simulink model "vhs_fpga_rx_to_sdram_time_share_agc"  (Simulink 7.1)
settings: Solver=FixedStepDiscrete  SolverMode=SingleTasking  StartTime=0.0  StopTime=inf  RelTol=1e-3
values from neighbouring files (symbols this model uses):
  N_FB_RX_frame = 390    [OFDM_Parameter.mat]
  Nfft = 64    [OFDM_Parameter.mat]
  Nguard = 16    [OFDM_Parameter.mat]
  Nofdm = 130    [OFDM_Parameter.mat]
libraries: xbsIndex_r4 x181, vhsadac_common_ob_fpgalib_v1_2_0 x17, misc_tools_fpgalib_v1_0_0 x2, rffe_fpgalib_v1_1_0 x1, rtdex_fpgalib_v1_1_0 x1
(part 2 of 2)

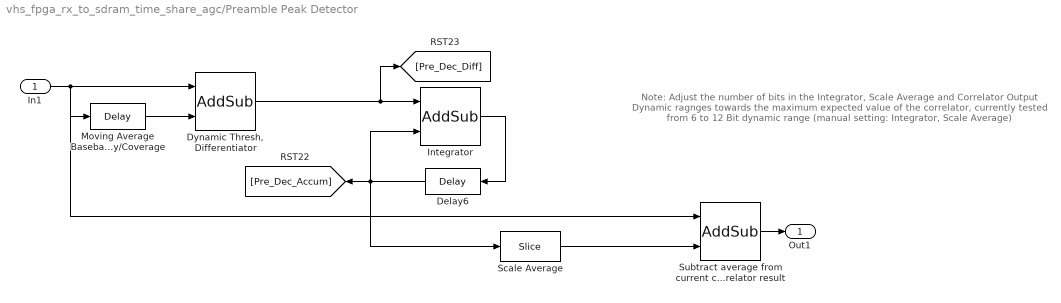
== system vhs_fpga_rx_to_sdram_time_share_agc/Preamble Peak Detector ==
  note: Note: Adjust the number of bits in the Integrator, Scale Average and Correlator Output Dynamic ragnges
      |  towards the maximum expected value of the correlator, currently tested from 6 to 12 Bit dynamic range
      |  (manual setting: Integrator, Scale Average)
  In1 : Inport
  Delay6 : xbsIndex_r4/Delay  Orientation=left  en=off  latency=1  dbl_ovrd=off  reg_retiming=off  block_type=delay
  "Dynamic Thresh, Differentiator" : xbsIndex_r4/AddSub  mode=Subtraction  use_carryin=off  use_carryout=off  en=off  latency=0  precision=Full  arith_type=Unsigned  n_bits=16  bin_pt=14  quantization=Truncate  overflow=Wrap  dbl_ovrd=off  use_behavioral_HDL=off  pipelined=off  use_rpm=on  hw_selection=Fabric  block_type=addsub
      settings: block_version=10.1.3
  Integrator : xbsIndex_r4/AddSub  mode=Addition  use_carryin=off  use_carryout=off  en=off  latency=0  precision=User Defined  arith_type="Signed  (2's comp)"  n_bits=23  bin_pt=0  quantization=Truncate  overflow=Saturate  dbl_ovrd=off  use_behavioral_HDL=off  pipelined=off  use_rpm=on  hw_selection=Fabric  block_type=addsub
      settings: block_version=10.1.3
  Moving Average Baseband (20MHz) Delay/Coverage : xbsIndex_r4/Delay  en=off  latency=32  dbl_ovrd=off  reg_retiming=off  block_type=delay
  Scale Average : xbsIndex_r4/Slice  nbits=16  boolean_output=off  mode=Upper Bit Location + Width  bit1=-7  base1=MSB of Input  bit0=0  base0=LSB of Input  dbl_ovrd=off  block_type=slice
      settings: infoedit="Extracts a given range of bits from each input sample and presents it at the output.  The output type is ordinarily unsigned with binary point at zero, but can be Boolean when the slice is one bit wide.<P><P>Hardware notes: In hardware this block costs nothing."  block_version=10.1.3
  Subtract average from current correlator result : xbsIndex_r4/AddSub  mode=Subtraction  use_carryin=off  use_carryout=off  en=off  latency=0  precision=Full  arith_type=Unsigned  n_bits=16  bin_pt=14  quantization=Truncate  overflow=Wrap  dbl_ovrd=off  use_behavioral_HDL=off  pipelined=off  use_rpm=on  hw_selection=Fabric  block_type=addsub
      settings: block_version=10.1.3
  Out1 : Outport
  wires:
  Moving Average Baseband (20MHz) Delay/Coverage/1 -> "Dynamic Thresh, Differentiator"/2
  "Dynamic Thresh, Differentiator"/1 -> Integrator/1, [Pre_Dec_Diff]
  Integrator/1 -> Delay6/1
  Delay6/1 -> Integrator/2, [Pre_Dec_Accum], Scale Average/1
  Scale Average/1 -> Subtract average from current correlator result/2
  In1/1 -> Moving Average Baseband (20MHz) Delay/Coverage/1, Subtract average from current correlator result/1, "Dynamic Thresh, Differentiator"/1
  Subtract average from current correlator result/1 -> Out1/1

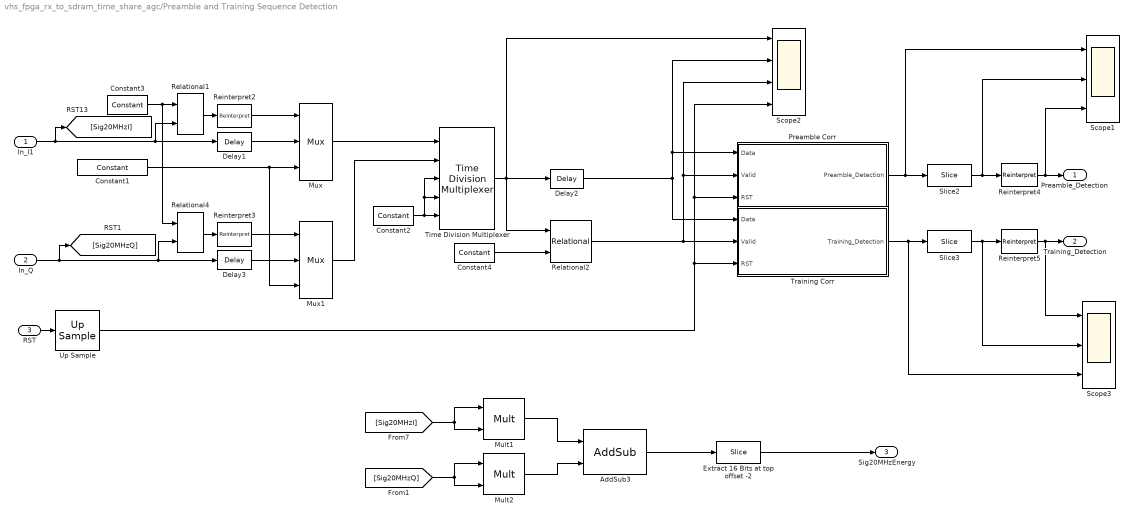
== system vhs_fpga_rx_to_sdram_time_share_agc/Preamble and Training Sequence Detection ==
  In_I1 : Inport  OutDataType=sfix(16)  OutScaling=2^0
  In_Q : Inport  Port=2  OutDataType=sfix(16)  OutScaling=2^0
  RST : Inport  Port=3  OutDataType=sfix(16)  OutScaling=2^0
  "   Extract 16 Bits at top offset -2" : xbsIndex_r4/Slice  nbits=16  boolean_output=off  mode=Upper Bit Location + Width  bit1=-2  base1=MSB of Input  bit0=0  base0=LSB of Input  dbl_ovrd=off  block_type=slice
      settings: infoedit="Extracts a given range of bits from each input sample and presents it at the output.  The output type is ordinarily unsigned with binary point at zero, but can be Boolean when the slice is one bit wide.<P><P>Hardware notes: In hardware this block costs nothing."  block_version=10.1.3
  AddSub3 : xbsIndex_r4/AddSub  mode=Addition  use_carryin=off  use_carryout=off  en=off  latency=1  precision=Full  arith_type=Unsigned  n_bits=16  bin_pt=14  quantization=Truncate  overflow=Wrap  dbl_ovrd=off  use_behavioral_HDL=off  pipelined=off  use_rpm=on  hw_selection=Fabric  block_type=addsub
      settings: block_version=10.1.3
  Constant1 : xbsIndex_r4/Constant  arith_type=Signed (2's comp)  const=1  n_bits=14  bin_pt=0  explicit_period=on  period=5  equ=P=C  opselect=C  inp2=PCIN>>17  opr=+  inp1=P  carry=CIN  dbl_ovrd=off  block_type=constant
  Constant2 : xbsIndex_r4/Constant  arith_type=Signed (2's comp)  const=0  n_bits=14  bin_pt=0  explicit_period=on  period=5  equ=P=C  opselect=C  inp2=PCIN>>17  opr=+  inp1=P  carry=CIN  dbl_ovrd=off  block_type=constant
  Constant3 : xbsIndex_r4/Constant  arith_type=Signed (2's comp)  const=0  n_bits=14  bin_pt=13  explicit_period=on  period=5  equ=P=C  opselect=C  inp2=PCIN>>17  opr=+  inp1=P  carry=CIN  dbl_ovrd=off  block_type=constant
  Constant4 : xbsIndex_r4/Constant  arith_type=Unsigned  const=0  n_bits=2  bin_pt=0  explicit_period=on  period=1  equ=P=C  opselect=C  inp2=PCIN>>17  opr=+  inp1=P  carry=CIN  dbl_ovrd=off  block_type=constant
  Delay1 : xbsIndex_r4/Delay  en=off  latency=1  dbl_ovrd=off  reg_retiming=off  block_type=delay
  Delay2 : xbsIndex_r4/Delay  en=off  latency=1  dbl_ovrd=off  reg_retiming=off  block_type=delay
  Delay3 : xbsIndex_r4/Delay  en=off  latency=1  dbl_ovrd=off  reg_retiming=off  block_type=delay
  Mult1 : xbsIndex_r4/Mult  precision=Full  arith_type="Signed  (2's comp)"  n_bits=16  bin_pt=14  quantization=Truncate  overflow=Wrap  en=off  latency=3  dbl_ovrd=off  use_behavioral_HDL=off  use_embedded=on  opt=Speed  optimum_pipeline=off  pipeline=on  use_rpm=on  placement_style=Triangular  block_type=mult
      settings: infoedit=Hardware notes: To use the internal pipeline stage of the dedicated multiplier you must select 'Pipeline for maximum performance'.  block_version=10.1.3
  Mult2 : xbsIndex_r4/Mult  precision=Full  arith_type="Signed  (2's comp)"  n_bits=16  bin_pt=14  quantization=Truncate  overflow=Wrap  en=off  latency=3  dbl_ovrd=off  use_behavioral_HDL=off  use_embedded=on  opt=Speed  optimum_pipeline=off  pipeline=on  use_rpm=on  placement_style=Triangular  block_type=mult
      settings: infoedit=Hardware notes: To use the internal pipeline stage of the dedicated multiplier you must select 'Pipeline for maximum performance'.  block_version=10.1.3
  Mux : xbsIndex_r4/Mux  inputs=2  en=off  latency=0  precision=Full  arith_type=Unsigned  n_bits=16  bin_pt=14  quantization=Truncate  overflow=Wrap  dbl_ovrd=off  block_type=mux
  Mux1 : xbsIndex_r4/Mux  inputs=2  en=off  latency=0  precision=Full  arith_type=Unsigned  n_bits=16  bin_pt=14  quantization=Truncate  overflow=Wrap  dbl_ovrd=off  block_type=mux
  Preamble Corr : Subsystem
  Reinterpret{2..5} (4 alike) : xbsIndex_r4/Reinterpret  force_arith_type=on  arith_type=Unsigned  force_bin_pt=on  bin_pt=0  block_type=reinterpret
      settings: infoedit="Changes signal type without altering the binary representation.   You can changed the signal between signed and unsigned, and relocate the binary point.<P><P>Hardware notes: In hardware this block costs nothing.<P><P>Example:  Suppose the input is 6 bits wide, signed, with 2 fractional bits, and the output is forced to unsigned with 0 fractional bits.  Then an input of -2.0 (1110.00 in binary 2's complement) becomes an output of 56 (111000 in binary)."  block_version=10.1.3
  Relational1 : xbsIndex_r4/Relational  mode=a=b  en=off  latency=1  dbl_ovrd=off  block_type=relational
      settings: block_version=10.1.3
  Relational2 : xbsIndex_r4/Relational  mode=a!=b  en=off  latency=1  dbl_ovrd=off  block_type=relational
      settings: block_version=10.1.3
  Relational4 : xbsIndex_r4/Relational  mode=a=b  en=off  latency=1  dbl_ovrd=off  block_type=relational
      settings: block_version=10.1.3
  Scope1 : Scope  NumInputPorts=3
      settings: YMin=-5~-5~-5  YMax=5~5~5  SaveName=ScopeData4  MaxDataPoints=500000  SampleInput=on
  Scope2 : Scope  NumInputPorts=4
      settings: YMin=-5~-5~-5~-5  YMax=5~5~5~5  SaveName=ScopeData3  MaxDataPoints=500000
  Scope3 : Scope  NumInputPorts=3
      settings: YMin=-5~-5~-5  YMax=5~5~5  SaveName=ScopeData5  MaxDataPoints=500000  SampleInput=on
  Slice2 : xbsIndex_r4/Slice  nbits=16  boolean_output=off  mode=Upper Bit Location + Width  bit1=-8  base1=MSB of Input  bit0=0  base0=LSB of Input  dbl_ovrd=off  block_type=slice
      settings: infoedit="Extracts a given range of bits from each input sample and presents it at the output.  The output type is ordinarily unsigned with binary point at zero, but can be Boolean when the slice is one bit wide.<P><P>Hardware notes: In hardware this block costs nothing."  block_version=10.1.3
  Slice3 : xbsIndex_r4/Slice  nbits=16  boolean_output=off  mode=Upper Bit Location + Width  bit1=-8  base1=MSB of Input  bit0=0  base0=LSB of Input  dbl_ovrd=off  block_type=slice
      settings: infoedit="Extracts a given range of bits from each input sample and presents it at the output.  The output type is ordinarily unsigned with binary point at zero, but can be Boolean when the slice is one bit wide.<P><P>Hardware notes: In hardware this block costs nothing."  block_version=10.1.3
  Time Division Multiplexer : xbsIndex_r4/Time Division Multiplexer  inputs=5  vin=off  dbl_ovrd=off  explicit_period=off  period=1  block_type=tdm
      settings: infoedit="Multiple inputs are sampled and  presented serially at the output."  block_version=10.1.3
  Training Corr : Subsystem
  Up Sample : xbsIndex_r4/Up Sample  sample_ratio=5  copy_samples=on  dbl_ovrd=off  block_type=usamp
      settings: infoedit="Up samples input data.  Inserted values  can be zeros or copies of the most recent input sample.<P><P>Hardware notes: No hardware is needed if inserted values are copies of the input sample; otherwise, a mux and single bit flip-flop are used."  block_version=10.1.3
  Preamble_Detection : Outport  OutDataType=sfix(16)  OutScaling=2^0
  Training_Detection : Outport  Port=2  OutDataType=sfix(16)  OutScaling=2^0
  Sig20MHzEnergy : Outport  Port=3  OutDataType=sfix(16)  OutScaling=2^0
  wires:
  Preamble Corr/1(Preamble_Detection) -> Slice2/1, Scope1/1
  Training Corr/1(Training_Detection) -> Slice3/1, Scope3/3
  Time Division Multiplexer/1 -> Delay2/1, Scope2/1, Relational2/1
  Constant2/1 -> Time Division Multiplexer/5, Time Division Multiplexer/3, Time Division Multiplexer/4
  In_Q/1 -> Relational4/2, Delay3/1, [Sig20MHzQ]
  In_I1/1 -> Relational1/2, Delay1/1, [Sig20MHzI]
  Constant4/1 -> Relational2/2
  RST/1 -> Up Sample/1
  Delay2/1 -> Training Corr/1(Data), Preamble Corr/1(Data), Scope2/2
  Up Sample/1 -> Training Corr/3(RST), Preamble Corr/3(RST), Scope2/4
  Relational2/1 -> Training Corr/2(Valid), Preamble Corr/2(Valid), Scope2/3
  Mux/1 -> Time Division Multiplexer/1
  Mux1/1 -> Time Division Multiplexer/2
  Constant1/1 -> Mux/3, Mux1/3
  Constant3/1 -> Relational1/1, Relational4/1
  Relational1/1 -> Reinterpret2/1
  Relational4/1 -> Reinterpret3/1
  Reinterpret2/1 -> Mux/1
  Reinterpret3/1 -> Mux1/1
  Delay1/1 -> Mux/2
  Delay3/1 -> Mux1/2
  Slice2/1 -> Reinterpret4/1, Scope1/2
  Slice3/1 -> Reinterpret5/1, Scope3/2
  Reinterpret4/1 -> Preamble_Detection/1, Scope1/3
  Reinterpret5/1 -> Training_Detection/1, Scope3/1
  [Sig20MHzI] -> Mult1/1, Mult1/2
  [Sig20MHzQ] -> Mult2/2, Mult2/1
  Mult1/1 -> AddSub3/1
  Mult2/1 -> AddSub3/2
  AddSub3/1 -> "   Extract 16 Bits at top offset -2"/1
  "   Extract 16 Bits at top offset -2"/1 -> Sig20MHzEnergy/1

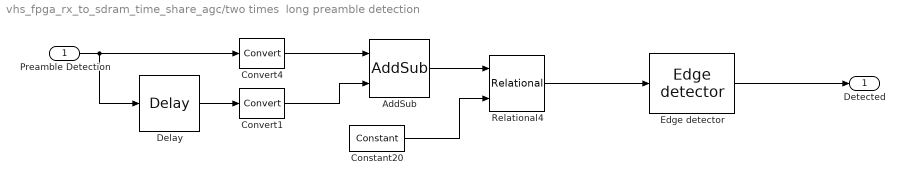
== system vhs_fpga_rx_to_sdram_time_share_agc/two times  long preamble detection ==
  Preamble Detection : Inport  OutDataType=sfix(16)  OutScaling=2^0
  AddSub : xbsIndex_r4/AddSub  mode=Addition  use_carryin=off  use_carryout=off  en=off  latency=0  precision=Full  arith_type=Unsigned  n_bits=16  bin_pt=14  quantization=Truncate  overflow=Wrap  dbl_ovrd=off  use_behavioral_HDL=off  pipelined=off  use_rpm=on  hw_selection=Fabric  block_type=addsub
      settings: block_version=9.2.00
  Constant20 : xbsIndex_r4/Constant  arith_type=Signed (2's comp)  const=2  n_bits=3  bin_pt=0  explicit_period=on  period=5  equ=P=C  opselect=C  inp2=PCIN>>17  opr=+  inp1=P  carry=CIN  dbl_ovrd=off  block_type=constant
      settings: block_version=9.2.00
  Convert1 : xbsIndex_r4/Convert  arith_type="Signed  (2's comp)"  n_bits=3  bin_pt=0  quantization=Truncate  overflow=Wrap  latency=0  dbl_ovrd=off  pipeline=off  block_type=convert
      settings: block_version=9.2.00
  Convert4 : xbsIndex_r4/Convert  arith_type="Signed  (2's comp)"  n_bits=3  bin_pt=0  quantization=Truncate  overflow=Wrap  latency=0  dbl_ovrd=off  pipeline=off  block_type=convert
      settings: block_version=9.2.00
  Delay : xbsIndex_r4/Delay  en=off  latency=(Nfft+Nguard)  dbl_ovrd=off  reg_retiming=off  block_type=delay
      settings: block_version=9.2.00
  Edge detector : misc_tools_fpgalib_v1_0_0/Edge detector  Tag=LYR_FPGA_MISC_EDGE_DETECTOR  Description=Lyrtech block  SystemSampleTime=-1  edge_detect=Rising  and_latency=0
  Relational4 : xbsIndex_r4/Relational  mode=a=b  en=off  latency=1  dbl_ovrd=off  block_type=relational
      settings: block_version=9.2.00
  Detected : Outport  OutDataType=sfix(16)  OutScaling=2^0
  wires:
  AddSub/1 -> Relational4/1
  Constant20/1 -> Relational4/2
  Convert4/1 -> AddSub/1
  Preamble Detection/1 -> Convert4/1, Delay/1
  Convert1/1 -> AddSub/2
  Delay/1 -> Convert1/1
  Relational4/1 -> Edge detector/1
  Edge detector/1 -> Detected/1

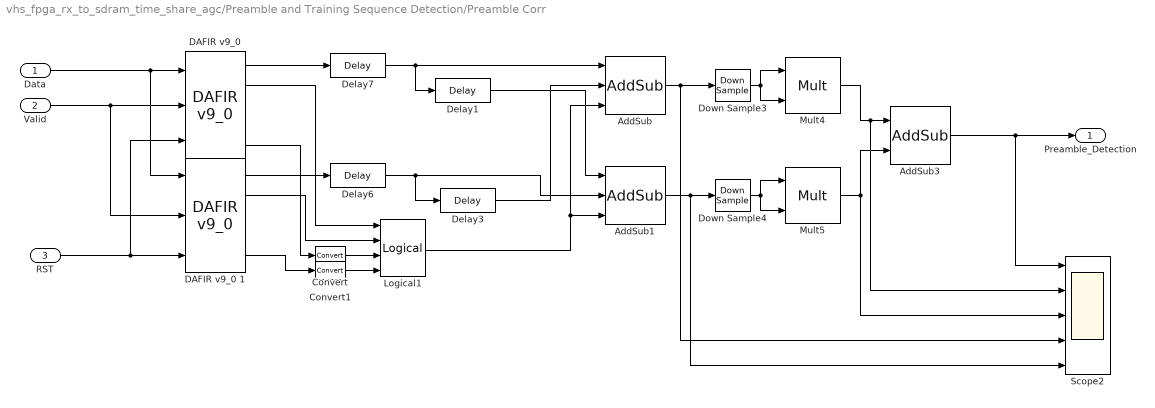
== system vhs_fpga_rx_to_sdram_time_share_agc/Preamble and Training Sequence Detection/Preamble Corr ==
  Data : Inport  OutDataType=sfix(16)  OutScaling=2^0
  Valid : Inport  Port=2  OutDataType=sfix(16)  OutScaling=2^0
  RST : Inport  Port=3  OutDataType=sfix(16)  OutScaling=2^0
  AddSub : xbsIndex_r4/AddSub  mode=Addition  use_carryin=off  use_carryout=off  en=on  latency=1  precision=Full  arith_type=Unsigned  n_bits=16  bin_pt=14  quantization=Truncate  overflow=Wrap  dbl_ovrd=off  use_behavioral_HDL=off  pipelined=off  use_rpm=on  hw_selection=Fabric  block_type=addsub
      settings: block_version=10.1.3
  AddSub1 : xbsIndex_r4/AddSub  mode=Subtraction  use_carryin=off  use_carryout=off  en=on  latency=1  precision=Full  arith_type=Unsigned  n_bits=16  bin_pt=14  quantization=Truncate  overflow=Wrap  dbl_ovrd=off  use_behavioral_HDL=off  pipelined=off  use_rpm=on  hw_selection=Fabric  block_type=addsub
      settings: block_version=10.1.3
  AddSub3 : xbsIndex_r4/AddSub  mode=Addition  use_carryin=off  use_carryout=off  en=off  latency=1  precision=Full  arith_type=Unsigned  n_bits=16  bin_pt=14  quantization=Truncate  overflow=Wrap  dbl_ovrd=off  use_behavioral_HDL=off  pipelined=off  use_rpm=on  hw_selection=Fabric  block_type=addsub
      settings: block_version=10.1.3
  Convert : xbsIndex_r4/Convert  arith_type=Boolean  n_bits=16  bin_pt=14  quantization=Truncate  overflow=Wrap  latency=0  dbl_ovrd=off  pipeline=off  block_type=convert
      settings: block_version=10.1.3
  Convert1 : xbsIndex_r4/Convert  arith_type=Boolean  n_bits=16  bin_pt=14  quantization=Truncate  overflow=Wrap  latency=0  dbl_ovrd=off  pipeline=off  block_type=convert
      settings: block_version=10.1.3
  "DAFIR v9_0 " : xbsIndex_r4/DAFIR v9_0   coef=2^8 * real( conj([(longPreamble_time(end:-1:end-Nguard+1)) (longPreamble_time(end:-1:1))]) )  structure=Inferred from Coefficients  coef_n_bits=10  coef_bin_pt=0  over_sample=1  reload=off  valids=on  rst=on  latency=11  num_channels=2  serial_input=on  polyphase_behavior="Single Rate:  sample in - sample out"  dbl_ovrd=off  explicit_period=off  period=1  use_isim=0  block_type=fir
      settings: infoedit="Hardware notes: Implemented using distributed arithmetic (DA).  The hardware over sampling rate determines the degree of parallelism.  A rate of one produces a fully parallel DA filter.  A rate of n (resp., n+1) for an n-bit input signal produces a fully serial implementation for a non-symmetric (resp., symmetric) impulse response.  Intermediate values produce implementations with intermediate levels of parallelism."  block_version=10.1.3
  DAFIR v9_0 1 : xbsIndex_r4/DAFIR v9_0   coef=2^8 * imag( conj([(longPreamble_time(end:-1:end-Nguard+1)) (longPreamble_time(end:-1:1))]) )  structure=Inferred from Coefficients  coef_n_bits=10  coef_bin_pt=0  over_sample=1  reload=off  valids=on  rst=on  latency=11  num_channels=2  serial_input=on  polyphase_behavior="Single Rate:  sample in - sample out"  dbl_ovrd=off  explicit_period=off  period=1  use_isim=0  block_type=fir
      settings: infoedit="Hardware notes: Implemented using distributed arithmetic (DA).  The hardware over sampling rate determines the degree of parallelism.  A rate of one produces a fully parallel DA filter.  A rate of n (resp., n+1) for an n-bit input signal produces a fully serial implementation for a non-symmetric (resp., symmetric) impulse response.  Intermediate values produce implementations with intermediate levels of parallelism."  block_version=10.1.3
  Delay{1,3,6..7} (4 alike) : xbsIndex_r4/Delay  en=off  latency=1  dbl_ovrd=off  reg_retiming=off  block_type=delay
  Down Sample3 : xbsIndex_r4/Down Sample  sample_ratio=5  sample_phase="Last Value of Frame  (most efficient)"  en=off  latency=1  dbl_ovrd=off  block_type=dsamp
      settings: block_version=10.1.3
  Down Sample4 : xbsIndex_r4/Down Sample  sample_ratio=5  sample_phase="Last Value of Frame  (most efficient)"  en=off  latency=1  dbl_ovrd=off  block_type=dsamp
      settings: block_version=10.1.3
  Logical1 : xbsIndex_r4/Logical  logical_function=AND  inputs=4  en=off  latency=1  precision=Full  arith_type=Unsigned  n_bits=16  bin_pt=0  align_bp=on  dbl_ovrd=off  block_type=logical
  Mult4 : xbsIndex_r4/Mult  precision=Full  arith_type="Signed  (2's comp)"  n_bits=16  bin_pt=14  quantization=Truncate  overflow=Wrap  en=off  latency=3  dbl_ovrd=off  use_behavioral_HDL=off  use_embedded=on  opt=Speed  optimum_pipeline=off  pipeline=on  use_rpm=on  placement_style=Triangular  block_type=mult
      settings: infoedit=Hardware notes: To use the internal pipeline stage of the dedicated multiplier you must select 'Pipeline for maximum performance'.  block_version=10.1.3
  Mult5 : xbsIndex_r4/Mult  precision=Full  arith_type="Signed  (2's comp)"  n_bits=16  bin_pt=14  quantization=Truncate  overflow=Wrap  en=off  latency=3  dbl_ovrd=off  use_behavioral_HDL=off  use_embedded=on  opt=Speed  optimum_pipeline=off  pipeline=on  use_rpm=on  placement_style=Triangular  block_type=mult
      settings: infoedit=Hardware notes: To use the internal pipeline stage of the dedicated multiplier you must select 'Pipeline for maximum performance'.  block_version=10.1.3
  Scope2 : Scope  NumInputPorts=5
      settings: YMin=-5~-5~-5~-5~-5  YMax=5~5~5~5~5  MaxDataPoints=500000
  Preamble_Detection : Outport  OutDataType=sfix(16)  OutScaling=2^0
  wires:
  "DAFIR v9_0 "/2 -> Logical1/1
  DAFIR v9_0 1/2 -> Logical1/2
  "DAFIR v9_0 "/1 -> Delay7/1
  DAFIR v9_0 1/1 -> Delay6/1
  Delay7/1 -> Delay1/1, AddSub/1
  Delay6/1 -> Delay3/1, AddSub1/2
  Delay3/1 -> AddSub/2
  Logical1/1 -> AddSub1/3, AddSub/3
  "DAFIR v9_0 "/5 -> Convert/1
  DAFIR v9_0 1/5 -> Convert1/1
  Convert/1 -> Logical1/3
  Convert1/1 -> Logical1/4
  Valid/1 -> DAFIR v9_0 1/2, "DAFIR v9_0 "/2
  Data/1 -> "DAFIR v9_0 "/1, DAFIR v9_0 1/1
  RST/1 -> "DAFIR v9_0 "/3, DAFIR v9_0 1/3
  Delay1/1 -> AddSub1/1
  AddSub3/1 -> Preamble_Detection/1, Scope2/1
  AddSub/1 -> Scope2/4, Down Sample3/1
  AddSub1/1 -> Down Sample4/1, Scope2/5
  Down Sample3/1 -> Mult4/1, Mult4/2
  Down Sample4/1 -> Mult5/1, Mult5/2
  Mult4/1 -> AddSub3/1, Scope2/2
  Mult5/1 -> AddSub3/2, Scope2/3

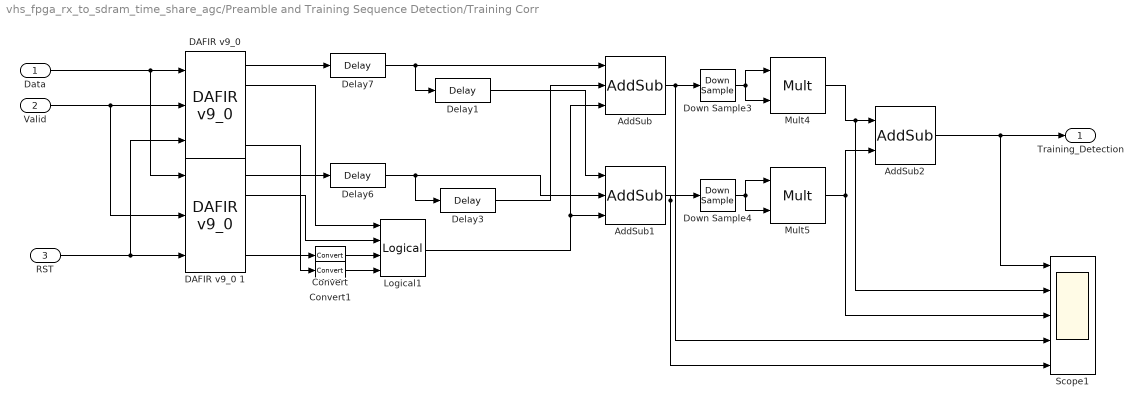
== system vhs_fpga_rx_to_sdram_time_share_agc/Preamble and Training Sequence Detection/Training Corr ==
  Data : Inport  OutDataType=sfix(16)  OutScaling=2^0
  Valid : Inport  Port=2  OutDataType=sfix(16)  OutScaling=2^0
  RST : Inport  Port=3  OutDataType=sfix(16)  OutScaling=2^0
  AddSub : xbsIndex_r4/AddSub  mode=Addition  use_carryin=off  use_carryout=off  en=on  latency=1  precision=Full  arith_type=Unsigned  n_bits=16  bin_pt=14  quantization=Truncate  overflow=Wrap  dbl_ovrd=off  use_behavioral_HDL=off  pipelined=off  use_rpm=on  hw_selection=Fabric  block_type=addsub
      settings: block_version=10.1.3
  AddSub1 : xbsIndex_r4/AddSub  mode=Subtraction  use_carryin=off  use_carryout=off  en=on  latency=1  precision=Full  arith_type=Unsigned  n_bits=16  bin_pt=14  quantization=Truncate  overflow=Wrap  dbl_ovrd=off  use_behavioral_HDL=off  pipelined=off  use_rpm=on  hw_selection=Fabric  block_type=addsub
      settings: block_version=10.1.3
  AddSub2 : xbsIndex_r4/AddSub  mode=Addition  use_carryin=off  use_carryout=off  en=off  latency=1  precision=Full  arith_type=Unsigned  n_bits=16  bin_pt=14  quantization=Truncate  overflow=Wrap  dbl_ovrd=off  use_behavioral_HDL=off  pipelined=off  use_rpm=on  hw_selection=Fabric  block_type=addsub
      settings: block_version=10.1.3
  Convert : xbsIndex_r4/Convert  arith_type=Boolean  n_bits=16  bin_pt=14  quantization=Truncate  overflow=Wrap  latency=0  dbl_ovrd=off  pipeline=off  block_type=convert
      settings: block_version=10.1.3
  Convert1 : xbsIndex_r4/Convert  arith_type=Boolean  n_bits=16  bin_pt=14  quantization=Truncate  overflow=Wrap  latency=0  dbl_ovrd=off  pipeline=off  block_type=convert
      settings: block_version=10.1.3
  "DAFIR v9_0 " : xbsIndex_r4/DAFIR v9_0   coef=2^7 * real( conj([(training_time(end:-1:end-Nguard+1)) (training_time(end:-1:1))]) )  structure=Inferred from Coefficients  coef_n_bits=10  coef_bin_pt=0  over_sample=1  reload=off  valids=on  rst=on  latency=11  num_channels=2  serial_input=on  polyphase_behavior="Single Rate:  sample in - sample out"  dbl_ovrd=off  explicit_period=off  period=1  use_isim=0  block_type=fir
      settings: infoedit="Hardware notes: Implemented using distributed arithmetic (DA).  The hardware over sampling rate determines the degree of parallelism.  A rate of one produces a fully parallel DA filter.  A rate of n (resp., n+1) for an n-bit input signal produces a fully serial implementation for a non-symmetric (resp., symmetric) impulse response.  Intermediate values produce implementations with intermediate levels of parallelism."  block_version=10.1.3
  DAFIR v9_0 1 : xbsIndex_r4/DAFIR v9_0   coef=2^7 * imag( conj([(training_time(end:-1:end-Nguard+1)) (training_time(end:-1:1))]) )  structure=Inferred from Coefficients  coef_n_bits=10  coef_bin_pt=0  over_sample=1  reload=off  valids=on  rst=on  latency=11  num_channels=2  serial_input=on  polyphase_behavior="Single Rate:  sample in - sample out"  dbl_ovrd=off  explicit_period=off  period=1  use_isim=0  block_type=fir
      settings: infoedit="Hardware notes: Implemented using distributed arithmetic (DA).  The hardware over sampling rate determines the degree of parallelism.  A rate of one produces a fully parallel DA filter.  A rate of n (resp., n+1) for an n-bit input signal produces a fully serial implementation for a non-symmetric (resp., symmetric) impulse response.  Intermediate values produce implementations with intermediate levels of parallelism."  block_version=10.1.3
  Delay{1,3,6..7} (4 alike) : xbsIndex_r4/Delay  en=off  latency=1  dbl_ovrd=off  reg_retiming=off  block_type=delay
  Down Sample3 : xbsIndex_r4/Down Sample  sample_ratio=5  sample_phase="Last Value of Frame  (most efficient)"  en=off  latency=1  dbl_ovrd=off  block_type=dsamp
      settings: block_version=10.1.3
  Down Sample4 : xbsIndex_r4/Down Sample  sample_ratio=5  sample_phase="Last Value of Frame  (most efficient)"  en=off  latency=1  dbl_ovrd=off  block_type=dsamp
      settings: block_version=10.1.3
  Logical1 : xbsIndex_r4/Logical  logical_function=AND  inputs=4  en=off  latency=1  precision=Full  arith_type=Unsigned  n_bits=16  bin_pt=0  align_bp=on  dbl_ovrd=off  block_type=logical
  Mult4 : xbsIndex_r4/Mult  precision=Full  arith_type="Signed  (2's comp)"  n_bits=16  bin_pt=14  quantization=Truncate  overflow=Wrap  en=off  latency=3  dbl_ovrd=off  use_behavioral_HDL=off  use_embedded=on  opt=Speed  optimum_pipeline=off  pipeline=on  use_rpm=on  placement_style=Triangular  block_type=mult
      settings: infoedit=Hardware notes: To use the internal pipeline stage of the dedicated multiplier you must select 'Pipeline for maximum performance'.  block_version=10.1.3
  Mult5 : xbsIndex_r4/Mult  precision=Full  arith_type="Signed  (2's comp)"  n_bits=16  bin_pt=14  quantization=Truncate  overflow=Wrap  en=off  latency=3  dbl_ovrd=off  use_behavioral_HDL=off  use_embedded=on  opt=Speed  optimum_pipeline=off  pipeline=on  use_rpm=on  placement_style=Triangular  block_type=mult
      settings: infoedit=Hardware notes: To use the internal pipeline stage of the dedicated multiplier you must select 'Pipeline for maximum performance'.  block_version=10.1.3
  Scope1 : Scope  NumInputPorts=5
      settings: YMin=-5~-5~-5~-5~-5  YMax=5~5~5~5~5  SaveName=ScopeData7  MaxDataPoints=500000
  Training_Detection : Outport  OutDataType=sfix(16)  OutScaling=2^0
  wires:
  "DAFIR v9_0 "/2 -> Logical1/1
  DAFIR v9_0 1/2 -> Logical1/2
  "DAFIR v9_0 "/1 -> Delay7/1
  DAFIR v9_0 1/1 -> Delay6/1
  Delay7/1 -> Delay1/1, AddSub/1
  Delay6/1 -> Delay3/1, AddSub1/2
  Delay3/1 -> AddSub/2
  Logical1/1 -> AddSub1/3, AddSub/3
  "DAFIR v9_0 "/5 -> Convert/1
  DAFIR v9_0 1/5 -> Convert1/1
  Convert/1 -> Logical1/3
  Convert1/1 -> Logical1/4
  Valid/1 -> DAFIR v9_0 1/2, "DAFIR v9_0 "/2
  Data/1 -> "DAFIR v9_0 "/1, DAFIR v9_0 1/1
  RST/1 -> "DAFIR v9_0 "/3, DAFIR v9_0 1/3
  Delay1/1 -> AddSub1/1
  AddSub2/1 -> Scope1/1, Training_Detection/1
  AddSub/1 -> Scope1/4, Down Sample3/1
  AddSub1/1 -> Scope1/5, Down Sample4/1
  Down Sample3/1 -> Mult4/1, Mult4/2
  Down Sample4/1 -> Mult5/1, Mult5/2
  Mult4/1 -> AddSub2/1, Scope1/2
  Mult5/1 -> AddSub2/2, Scope1/3
